simulink model "PendulumPID_Control"  (R2018b)
settings: Solver=VariableStepAuto  StartTime=0.0  StopTime=10.0  RelTol=1e-3
settings Model: Creator=Seko  LastModifiedBy=Seko

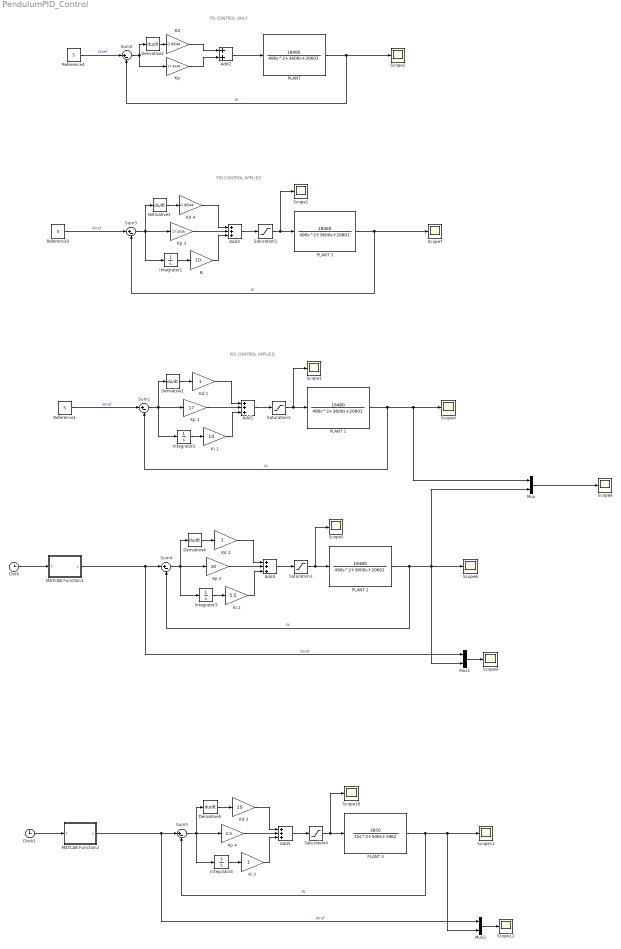
== system PendulumPID_Control ==
  note: PID CONTROL APPLIED
  note: PD CONTROL ONLY
  note: PID CONTROL APPLIED
  Add{1,3..5} (4 alike) : Sum  Inputs=+++
  Add2 : Sum
  Clock : Clock
  Clock1 : Clock
  Derivative{1..5} (5 alike) : Derivative
  Integrator{1..4} (4 alike) : Integrator
  "Kd " : Gain  Gain=0.9644
  Kd 1 : Gain
  Kd 2 : Gain
  Kd 3 : Gain  Gain=10
  Kd 4 : Gain  Gain=0.9644
  "Ki " : Gain  Gain=10
  Ki 1 : Gain  Gain=10
  Ki 2 : Gain  Gain=5.5
  Ki 3 : Gain
  "Kp " : Gain  Gain=17.4546
  Kp 1 : Gain  Gain=17
  Kp 2 : Gain  Gain=30
  Kp 3 : Gain  Gain=17.4546
  Kp 4 : Gain  Gain=2.5
  MATLAB Function1 : MATLAB Function  TreatAsAtomicUnit=on
  MATLAB Function2 : MATLAB Function  TreatAsAtomicUnit=on
  Mux : Mux  Inputs=2
  Mux1 : Mux  Inputs=2
  Mux2 : Mux  Inputs=2
  PLANT {,1..3} (4 alike) : TransferFcn  Numerator=[18480]  Denominator=[490 3600 20601]
  PLANT 4 : TransferFcn  Numerator=[3850]  Denominator=[15 500 1962]
  Reference1 : Constant  Value=5
  Reference3 : Constant  Value=5
  Reference4 : Constant  Value=5
  Saturation{1..4} (4 alike) : Saturate  UpperLimit=6  LowerLimit=-6
  Scope{1..12} (12 alike) : Scope
  Sum{1..5} (5 alike) : Sum  Inputs=|+-
  wires:
  Sum2/1 -> Derivative2/1, "Kp "/1
  "Kd "/1 -> Add2/1
  "Kp "/1 -> Add2/2
  Derivative2/1 -> "Kd "/1
  "PLANT "/1 -> Sum2/2, Scope2/1  "W"
  Add2/1 -> "PLANT "/1
  Reference4/1 -> Sum2/1  "Wref"
  PLANT 3/1 -> Scope7/1, Sum3/2  "W"
  Kp 3/1 -> Add3/2
  Derivative3/1 -> Kd 4/1
  Sum3/1 -> Derivative3/1, Integrator1/1, Kp 3/1
  Reference3/1 -> Sum3/1  "Wref"
  Kd 4/1 -> Add3/1
  Integrator1/1 -> "Ki "/1
  "Ki "/1 -> Add3/3
  Clock/1 -> MATLAB Function1/1(t)
  Add3/1 -> Saturation1/1
  Saturation1/1 -> Scope1/1, PLANT 3/1
  Ki 1/1 -> Add1/3
  Saturation2/1 -> Scope3/1, PLANT 1/1
  Add1/1 -> Saturation2/1
  Integrator2/1 -> Ki 1/1
  Kd 1/1 -> Add1/1
  PLANT 1/1 -> Mux/1, Scope4/1, Sum1/2  "W"
  Reference1/1 -> Sum1/1  "Wref"
  Sum1/1 -> Derivative1/1, Integrator2/1, Kp 1/1
  Kp 1/1 -> Add1/2
  Derivative1/1 -> Kd 1/1
  Kp 2/1 -> Add4/2
  Derivative4/1 -> Kd 2/1
  Sum4/1 -> Derivative4/1, Integrator3/1, Kp 2/1
  Add4/1 -> Saturation3/1
  Kd 2/1 -> Add4/1
  Integrator3/1 -> Ki 2/1
  PLANT 2/1 -> Mux1/2, Mux/2, Scope6/1, Sum4/2  "W"
  Saturation3/1 -> Scope5/1, PLANT 2/1
  Ki 2/1 -> Add4/3
  MATLAB Function1/1(y) -> Mux1/1, Sum4/1  "Wref"
  Mux/1 -> Scope8/1
  Mux1/1 -> Scope9/1
  MATLAB Function2/1(y) -> Mux2/1, Sum5/1  "Wref"
  Mux2/1 -> Scope12/1
  PLANT 4/1 -> Mux2/2, Scope11/1, Sum5/2  "W"
  Saturation4/1 -> Scope10/1, PLANT 4/1
  Integrator4/1 -> Ki 3/1
  Derivative5/1 -> Kd 3/1
  Kd 3/1 -> Add5/1
  Kp 4/1 -> Add5/2
  Sum5/1 -> Derivative5/1, Integrator4/1, Kp 4/1
  Ki 3/1 -> Add5/3
  Clock1/1 -> MATLAB Function2/1(t)
  Add5/1 -> Saturation4/1

== matlab function PendulumPID_Control/MATLAB Function1 ==
  data: t input; y output
function y = fcn(t)
f=1;
y=sin(2*pi*f*t);
end

== matlab function PendulumPID_Control/MATLAB Function2 ==
  data: t input; y output
function y = fcn(t)
f=1;
y=sin(2*pi*f*t);
end
